simulink model "Orbit"  (R2019b)
settings: Solver=FixedStepAuto  StartTime=0.0  StopTime=24  RelTol=1e-3
InitFcn:
  | load('BusDefinitions.mat')
model workspace (MAT data in the model file):
  MM = [1  1  1  1; 1  1  -1  -1; 1  -1  -1  1; 1  -1  1  -1]
  OrbitLab = 0.5
  SlowDownPeriod = 3
  Startlag = 1
  initDesc = 20
  p = 0.8638671875
  wDotBias = 9.242
values from neighbouring files (symbols this model uses):
  A = double(subs(A4disc,9.81))    [loadDiscSys.m]
  At = A2by2    [KalmanGains.m]
  B = double(subs(B4disc,9.81))    [loadDiscSys.m]
  BMove = 11    [PrimeO.m]
  Bt = [0;-0.0624]    [KalmanGains.m]
  C = eye(2)    [KalmanGains.m]    (also in loadDiscSys.m = eye(4))
  commandZ = -1.5    [Commands.m]
  Ct = fsolve(hover,.05)    [BangBangCalculations.m]
  End = 13    [PrimeO.m]
  FMove = 9    [PrimeO.m]
  Ka = lqr(Aa,Ba,Qa,Ra)    [KalmanGains.m]
  KaI = Ka(1)/2    [Commands.m]
  Ke = lqr(Ae,Be,Qe,Re)    [KalmanGains.m]
  KeI = Ke(1)*1.5    [Commands.m]
  Kr = Kr    [KalmanGains.m]
  KrI = Kr(1)/4    [Commands.m]
  Kt = lqr(At,Bt,Qt,Rt)    [KalmanGains.m]
  KtI = Kt(1)/4    [Commands.m]
  LMove = 7    [PrimeO.m]
  R = eye(4)*.001    [KalmanCosts.m]
  RMove = 5    [PrimeO.m]
  Rt = 11    [KalmanCosts.m]    (also in KalmanGains.m = 0.005)
  tSwitch = fsolve(Switch,.5)    [BangBangCalculations.m]
  tSwitchU = tSwitch+.30    [BangBangCalculations.m]
  w0 = fsolve(hover,300)    [BangBangCalculations.m]
  wD = fsolve(Down,300)    [BangBangCalculations.m]
  wU = fsolve(Up,300)    [BangBangCalculations.m]
undefined symbols (not defined in the file or in its folder): codertarget, DiscIntNeverNeededParam, Discrete, Dt, Time
libraries: simulink x14, ctrlSharedLib x2
settings Model: ExtModeTrigDuration=80  OrderedModelArguments=off  Creator=johnharry  LastModifiedBy=johnh
settings OptimizationCC: BlockReduction=off  DefaultParameterBehavior=Inlined  BufferReuse=off  PassReuseOutputArgsThreshold=0  MaxStackSize=64
settings DebuggingCC: ParameterTunabilityLossMsg=error  ArithmeticOperatorsInVariantConditions=warning
settings HardwareCC: ProdBitPerPointer=32  ProdBitPerSizeT=32  ProdBitPerPtrDiffT=32  ProdLargestAtomicInteger=Long  ProdWordSize=32  ProdHWDeviceType=ARM Compatible->ARM 9
settings SFSimCC: SimUseLocalCustomCode=off  MATLABDynamicMemAlloc=off
settings RTWCC: SystemTargetFile=ert.tlc  HardwareBoard=PARROT Mambo  TLCOptions="-aInlineSetEventsForThisBaseRateFcn=TLC_FALSE -aSuppressMultiTaskScheduler=TLC_FALSE   -aRateBasedStepFcn=1"  TemplateMakefile=ert_default_tmf  GenerateReport=on  RTWUseLocalCustomCode=off  Toolchain=Sourcery G++ Lite GNU Toolchain for Drones  LaunchReport=on
settings CodeAppCC: ForceParamTrailComments=on  OperatorAnnotations=on  StateflowObjectComments=on
settings ERTTargetCC: ERTCustomFileBanners=off  MatFileLogging=on  SupportContinuousTime=on  SupportNonInlinedSFcns=on  RemoveResetFunc=off  ModelStepFunctionPrototypeControlCompliant=off

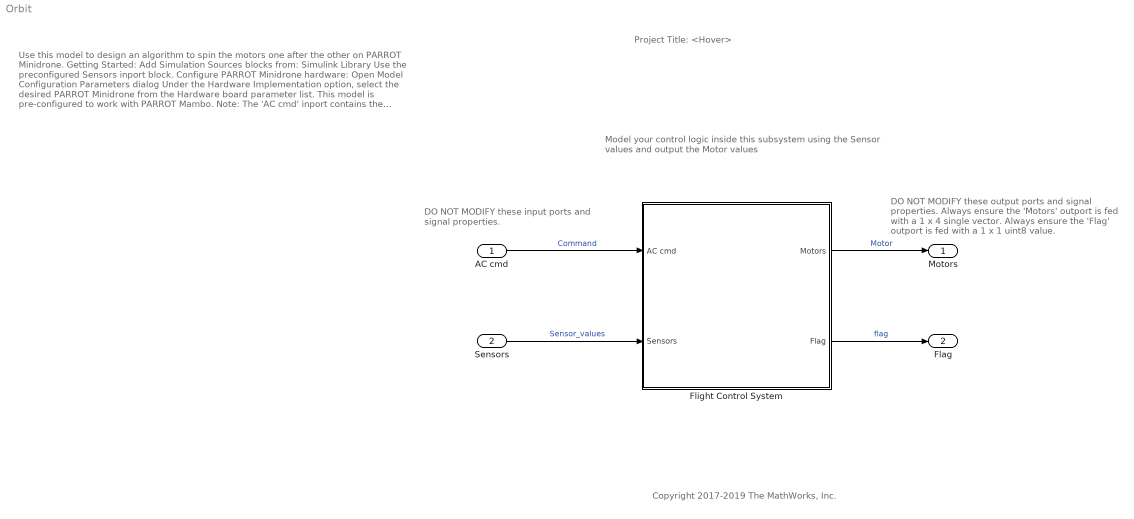
== system Orbit ==
  note: Model your control logic inside this subsystem
      | using the Sensor values and output the
      | Motor values
  note: DO NOT MODIFY these output ports
      | and signal properties.
      |
      |
      |
      | Always ensure the 'Motors' outport
      | is fed with a 1 x 4 single vector.
      |
      |
      |
      |
      |
      | Always ensure the 'Flag' outport is
      | fed with a 1 x 1 uint8 value.
  note: DO NOT MODIFY these input
      | ports and signal properties.
  note: Copyright 2017-2019 The MathWorks, Inc.
  note: Use this model to design an algorithm to spin the motors one
      | after the other on PARROT Minidrone.
      |
      | Getting Started:
      |
      | Add Simulation Sources blocks from:
      | Simulink Library
      | Use the preconfigured Sensors inport block.
      |
      | Configure PARROT Minidrone hardware:
      |
      | Open Model Configuration Parameters dialog
      |
      | Under the Hardware Implementation option, select the desired
      | PARROT Minidrone from the Hardware board parameter list.
      |
      | This model is pre-configured to work with PARROT Mambo.
      |
      | Note:
      |
      | The 'AC cmd' inport contains the position and orientation
      | reference signals information.
      | The 'Sensors' inport contains data from accelerometer,
      | gyroscope, ultrasonic, pressure and optical flow data.
      | The 'Flag' outport can be used to model an error condition
      | which stops the drone.
      | The 'Motors' outport is fed with the speed values of the 4 motors.
      | Learn more:
      |
      | Simulink Subsystem
      | Simulink Buses
  note: Project Title: <Hover>
  AC cmd : Inport  OutDataTypeStr=Bus: CommandBus  BusOutputAsStruct=on
  Sensors : Inport  Port=2  OutDataTypeStr=Bus: SensorsBus  BusOutputAsStruct=on
  Flight Control System : Subsystem  InitFcn=codertarget.parrot.internal.fcsSubsystemCallback(gcb);
  Motors : Outport  OutDataTypeStr=single  PortDimensions=[1 4]  VectorParamsAs1DForOutWhenUnconnected=off
  Flag : Outport  Port=2  OutDataTypeStr=uint8  PortDimensions=1  VectorParamsAs1DForOutWhenUnconnected=off
  wires:
  Flight Control System/1(Motors) -> Motors/1  "Motor"
  AC cmd/1 -> Flight Control System/1(AC cmd)  "Command"
  Sensors/1 -> Flight Control System/2(Sensors)  "Sensor_values"
  Flight Control System/2(Flag) -> Flag/1  "flag"

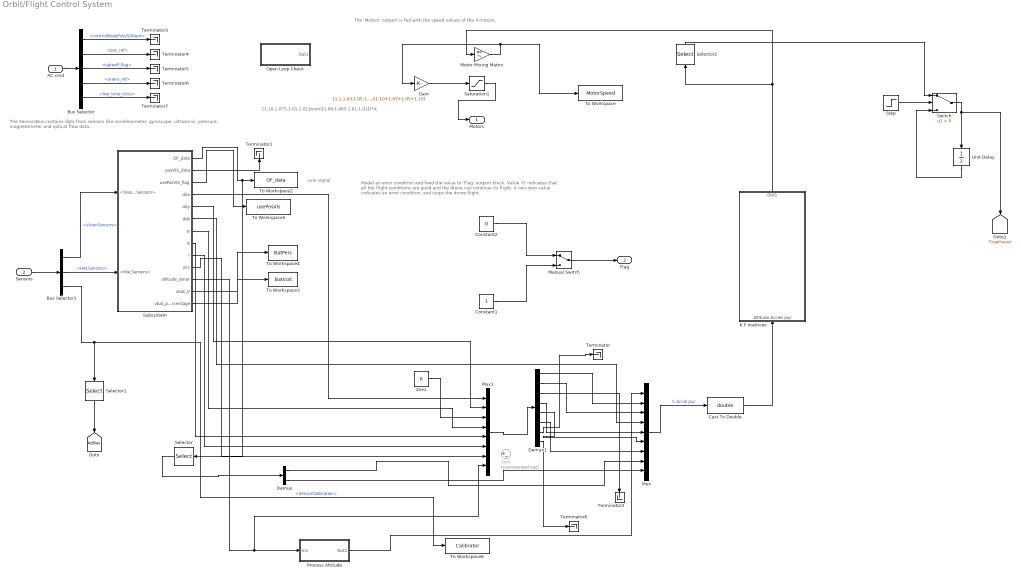
== system Orbit/Flight Control System ==
  note: [1.10,1.075,1.01,1.01]/sum([1.09,1.065,1.01,1.01])*4;
  note: uvw signal
  note: The 'Motors' outport is fed with the speed values of the 4 motors.
  note: Model an error condition and feed the value to 'Flag' outport block.
      | Value '0' indicates that all the flight conditions are good and the drone
      | can continue its flight.
      | A non-zero value indicates an error condition, and stops the drone
      | flight.
  note: The SensorsBus contains data from sensors like
      | accelerometer, gyroscope, ultrasonic, pressure,
      | magnetometer and optical flow data.
  AC cmd : Inport
  Sensors : Inport  Port=2
  Bus Selector : BusSelector  OutputSignals=controlModePosVSOrient,pos_ref,takeoff_flag,orient_ref,live_time_ticks
  Bus Selector1 : BusSelector  OutputSignals=VisionSensors,HALSensors,SensorCalibration
  Cast To Double : DataTypeConversion  OutDataTypeStr=double
  Constant1 : Constant  OutDataTypeStr=uint8
  Constant2 : Constant  Value=0  OutDataTypeStr=uint8
  Demux : Demux  Outputs=2
  Demux1 : Demux  Outputs=8
  Gain : Gain  Gain=[1.1,1.03,1.05,1.15].*4./(1.10+1.03+1.05+1.15)
  K F matrices : Subsystem
  Manual Switch : ManualSwitch
  Motor Mixing Matrix : Gain  Gain=MM  Multiplication=Matrix(K*u)
  Mux : Mux  Inputs=9
  Mux1 : Mux  Inputs=8
  Open Loop Check : Subsystem
  Process Altitude : Subsystem
  Saturation1 : Saturate  UpperLimit=500  LowerLimit=0  OutDataTypeStr=single
  Selector : Selector  InputPortWidth=3  IndexOptions=Index vector (dialog)  Indices=[1 2]  OutputSizes=1
  Selector1 : Selector  IndexOptions=Index vector (dialog)  Indices=3  OutputSizes=1
  Selector2 : Selector  InputPortWidth=4  IndexOptions=Index vector (dialog)  Indices=1  OutputSizes=1
  Step : Step  Time=tSwitch+tSwitchU+Startlag+OrbitLab  SampleTime=.005
  Subsystem : Subsystem
  Sum : Sum  Commented=on  Inputs=|+-
  Switch : Switch  Criteria=u2 > Threshold
  Terminator{,1..8} (9 alike) : Terminator
  To Workspace : ToWorkspace  VariableName=MotorSpeed  SaveFormat=Structure With Time  SampleTime=-1
  To Workspace2 : ToWorkspace  VariableName=OF_data  SaveFormat=Structure With Time  SampleTime=-1
  To Workspace3 : ToWorkspace  VariableName=BatVolt  SaveFormat=Structure With Time  SampleTime=-1
  To Workspace4 : ToWorkspace  VariableName=BatPerc  SaveFormat=Structure With Time  SampleTime=-1
  To Workspace5 : ToWorkspace  VariableName=usePosVis  SaveFormat=Structure With Time  SampleTime=-1
  To Workspace6 : ToWorkspace  VariableName=Calibrator  SaveFormat=Timeseries  SampleTime=-1
  Unit Delay : UnitDelay  SampleTime=-1  HasFrameUpgradeWarning=on
  Zero : Constant  Value=0  OutDataTypeStr=Inherit: Inherit via back propagation  SampleTime=.005
  Motors : Outport  VectorParamsAs1DForOutWhenUnconnected=off
  Flag : Outport  Port=2  VectorParamsAs1DForOutWhenUnconnected=off
  tag scope: AzBias=global, TrueHover=global
  wires:
  AC cmd/1 -> Bus Selector/1
  Sensors/1 -> Bus Selector1/1
  Bus Selector/1 -> Terminator3/1  "<controlModePosVSOrient>"
  Bus Selector/2 -> Terminator4/1  "<pos_ref>"
  Bus Selector/3 -> Terminator5/1  "<takeoff_flag>"
  Bus Selector/4 -> Terminator6/1  "<orient_ref>"
  Bus Selector/5 -> Terminator7/1  "<live_time_ticks>"
  Manual Switch/1 -> Flag/1
  Constant2/1 -> Manual Switch/1
  Constant1/1 -> Manual Switch/2
  Saturation1/1 -> Motors/1
  Bus Selector1/1 -> Subsystem/1(<VisionSensors>)  "<VisionSensors>"
  Bus Selector1/2 -> Subsystem/2(<HALSensors>)  "<HALSensors>"
  Bus Selector1/3 -> Selector1/1, To Workspace6/1  "<SensorCalibration>"
  Subsystem/1(OF_data) -> Selector/1, To Workspace2/1
  Subsystem/3(usePosVIS_flag) -> To Workspace5/1
  Subsystem/12(vbat_V) -> To Workspace3/1
  Subsystem/13(vbat_percentage) -> To Workspace4/1
  Subsystem/5(ddy) -> Mux1/2
  Subsystem/8(q) -> Mux1/5
  Subsystem/7(p) -> Mux1/4
  Subsystem/9(r) -> Mux1/6
  Subsystem/4(ddx) -> Mux1/1
  Mux/1 -> Cast To Double/1  "h Accel pqr"
  Subsystem/6(ddz) -> Mux/4
  Motor Mixing Matrix/1 -> Gain/1, To Workspace/1
  Subsystem/11(altitude_sonar) -> Mux1/8, Process Altitude/1(In1)
  K F matrices/1(Out1) -> Motor Mixing Matrix/1, Selector2/1
  Gain/1 -> Saturation1/1
  Cast To Double/1 -> K F matrices/1(Altitude Accels pqr)
  Selector/1 -> Demux/1
  Demux/1 -> Mux/8
  Demux/2 -> Mux/9
  Subsystem/10(prs) -> Mux1/7
  Mux1/1 -> Demux1/1
  Demux1/1 -> Mux/2
  Demux1/2 -> Mux/3
  Demux1/3 -> Terminator2/1
  Demux1/4 -> Mux/5
  Demux1/5 -> Mux/6
  Demux1/6 -> Mux/7
  Demux1/8 -> Terminator8/1
  Demux1/7 -> Terminator/1
  Subsystem/2(posVIS_data) -> Terminator1/1
  Zero/1 -> Mux1/3
  Selector1/1 -> [AzBias]
  Process Altitude/1(Out1) -> Mux/1
  Switch/1 -> [TrueHover], Unit Delay/1
  Selector2/1 -> Switch/1
  Unit Delay/1 -> Switch/3
  Step/1 -> Switch/2

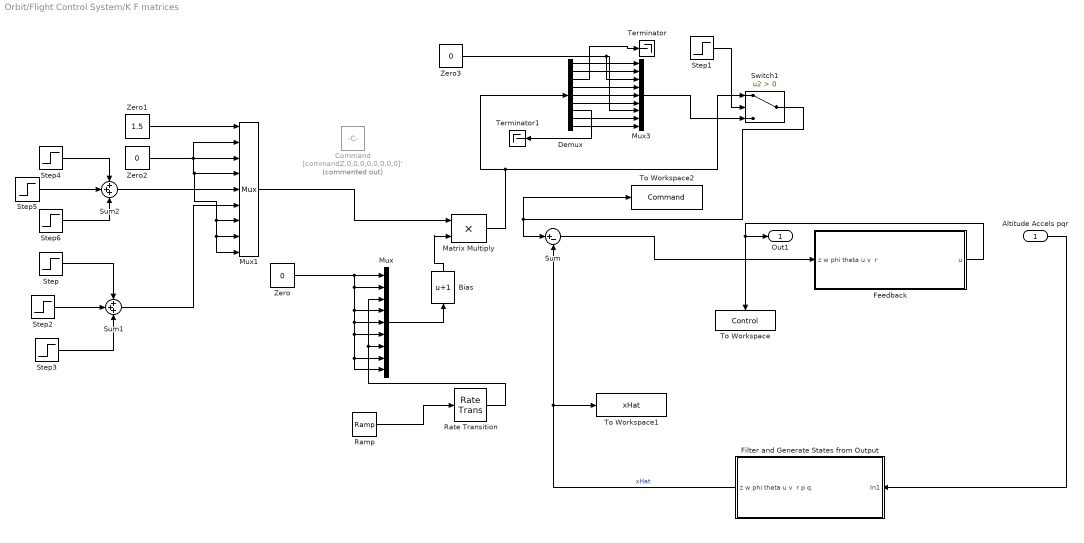
== system Orbit/Flight Control System/K F matrices ==
  Altitude Accels pqr : Inport
  Bias : Bias  Bias=1
  Command : Constant  Commented=on  Value=[commandZ,0,0,0,0,0,0,0,0]'  OutDataTypeStr=Inherit: Inherit via back propagation  SampleTime=.005
  Demux : Demux  Outputs=9
  Feedback : Subsystem
  Filter and Generate States from Output : Subsystem
  Matrix Multiply : Product
  Mux : Mux  Inputs=9
  Mux1 : Mux  Inputs=9
  Mux3 : Mux  Inputs=9
  Ramp : simulink/Sources/Ramp  slope=1/60  start=tSwitch+Startlag+tSwitchU+OrbitLab  InitialOutput=0
  Rate Transition : RateTransition  OutPortSampleTime=.005
  Step : Step  Time=RMove  After=.25  SampleTime=.005
  Step1 : Step  Time=initDesc-SlowDownPeriod  Before=1  After=-1  SampleTime=.005
  Step2 : Step  Time=LMove  After=-.5  SampleTime=.005
  Step3 : Step  Time=FMove  After=.25  SampleTime=.005
  Step4 : Step  Time=FMove  After=.25  SampleTime=.005
  Step5 : Step  Time=BMove  After=-.5  SampleTime=.005
  Step6 : Step  Time=End  After=.25  SampleTime=.005
  Sum : Sum  Inputs=|+-
  Sum1 : Sum  Inputs=+++
  Sum2 : Sum  Inputs=+++
  Switch1 : Switch  Criteria=u2 > Threshold
  Terminator : Terminator
  Terminator1 : Terminator
  To Workspace : ToWorkspace  VariableName=Control  SaveFormat=Structure With Time  SampleTime=-1
  To Workspace1 : ToWorkspace  VariableName=xHat  SaveFormat=Structure With Time  SampleTime=-1
  To Workspace2 : ToWorkspace  VariableName=Command  SaveFormat=Structure With Time  SampleTime=-1
  Zero : Constant  Value=0  OutDataTypeStr=Inherit: Inherit via back propagation  SampleTime=.005
  Zero1 : Constant  Value=1.5  OutDataTypeStr=Inherit: Inherit via back propagation  SampleTime=.005
  Zero2 : Constant  Value=0  OutDataTypeStr=Inherit: Inherit via back propagation  SampleTime=.005
  Zero3 : Constant  Value=0  OutDataTypeStr=Inherit: Inherit via back propagation  SampleTime=.005
  Out1 : Outport
  wires:
  Filter and Generate States from Output/1(z w phi theta u v  r p q) -> To Workspace1/1, Sum/2  "xHat"
  Feedback/1("u ") -> Out1/1, To Workspace/1
  Sum/1 -> Feedback/1(z w phi theta u v  r)
  Altitude Accels pqr/1 -> Filter and Generate States from Output/1(In1)
  Ramp/1 -> Rate Transition/1
  Rate Transition/1 -> Mux/3, Mux/7
  Zero/1 -> Mux/9, Mux/8, Mux/6, Mux/5, Mux/4, Mux/2, Mux/1
  Mux/1 -> Bias/1
  Bias/1 -> Matrix Multiply/2
  Matrix Multiply/1 -> Demux/1, Switch1/1
  Step1/1 -> Switch1/2
  Demux/1 -> Mux3/1
  Demux/2 -> Mux3/2
  Demux/9 -> Mux3/9
  Demux/8 -> Mux3/8
  Demux/7 -> Terminator1/1
  Demux/6 -> Mux3/6
  Demux/5 -> Mux3/5
  Demux/4 -> Mux3/4
  Mux3/1 -> Switch1/3
  Switch1/1 -> To Workspace2/1, Sum/1
  Zero3/1 -> Mux3/7, Mux3/3
  Demux/3 -> Terminator/1
  Zero1/1 -> Mux1/1
  Zero2/1 -> Mux1/8, Mux1/9, Mux1/7, Mux1/4, Mux1/3, Mux1/2
  Sum1/1 -> Mux1/6
  Sum2/1 -> Mux1/5
  Step3/1 -> Sum1/3
  Step2/1 -> Sum1/2
  Step/1 -> Sum1/1
  Step4/1 -> Sum2/1
  Step5/1 -> Sum2/2
  Step6/1 -> Sum2/3
  Mux1/1 -> Matrix Multiply/1

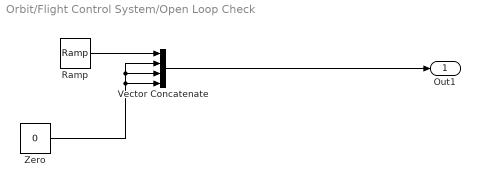
== system Orbit/Flight Control System/Open Loop Check ==
  Ramp : simulink/Sources/Ramp  slope=40  start=0  InitialOutput=0
  Vector Concatenate : Concatenate  NumInputs=4
  Zero : Constant  Value=0  OutDataTypeStr=Inherit: Inherit via back propagation
  Out1 : Outport
  wires:
  Vector Concatenate/1 -> Out1/1
  Zero/1 -> Vector Concatenate/4, Vector Concatenate/3, Vector Concatenate/2
  Ramp/1 -> Vector Concatenate/1

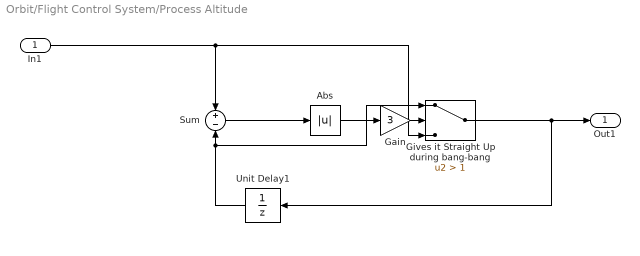
== system Orbit/Flight Control System/Process Altitude ==
  In1 : Inport  PortDimensions=1
  Abs : Abs
  Gain : Gain  Gain=3
  Gives it Straight Up during bang-bang : Switch  Criteria=u2 > Threshold  Threshold=1
  Sum : Sum  Inputs=+-
  Unit Delay1 : UnitDelay  SampleTime=-1  HasFrameUpgradeWarning=on
  Out1 : Outport  PortDimensions=1
  wires:
  In1/1 -> Gives it Straight Up during bang-bang/3, Sum/1
  Gives it Straight Up during bang-bang/1 -> Unit Delay1/1, Out1/1
  Unit Delay1/1 -> Gives it Straight Up during bang-bang/1, Sum/2
  Sum/1 -> Abs/1
  Abs/1 -> Gain/1
  Gain/1 -> Gives it Straight Up during bang-bang/2

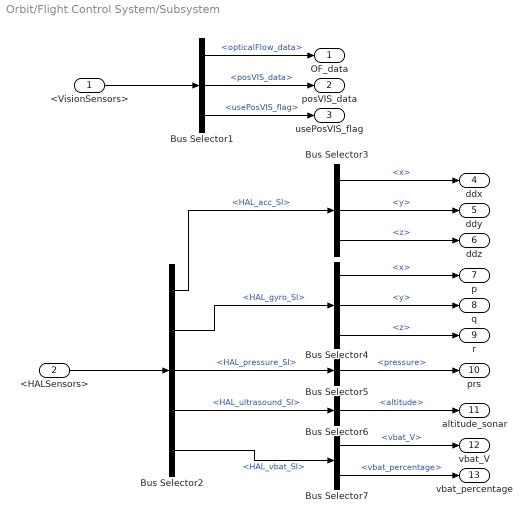
== system Orbit/Flight Control System/Subsystem ==
  <VisionSensors> : Inport
  <HALSensors> : Inport  Port=2
  Bus Selector1 : BusSelector  OutputSignals=opticalFlow_data,posVIS_data,usePosVIS_flag
  Bus Selector2 : BusSelector  OutputSignals=HAL_acc_SI,HAL_gyro_SI,HAL_pressure_SI,HAL_ultrasound_SI,HAL_vbat_SI
  Bus Selector3 : BusSelector  OutputSignals=x,y,z
  Bus Selector4 : BusSelector  OutputSignals=x,y,z
  Bus Selector5 : BusSelector  OutputSignals=pressure
  Bus Selector6 : BusSelector  OutputSignals=altitude
  Bus Selector7 : BusSelector  OutputSignals=vbat_V,vbat_percentage
  OF_data : Outport  VectorParamsAs1DForOutWhenUnconnected=off
  posVIS_data : Outport  Port=2  VectorParamsAs1DForOutWhenUnconnected=off
  usePosVIS_flag : Outport  Port=3  VectorParamsAs1DForOutWhenUnconnected=off
  ddx : Outport  Port=4  VectorParamsAs1DForOutWhenUnconnected=off
  ddy : Outport  Port=5  VectorParamsAs1DForOutWhenUnconnected=off
  ddz : Outport  Port=6  VectorParamsAs1DForOutWhenUnconnected=off
  p : Outport  Port=7  VectorParamsAs1DForOutWhenUnconnected=off
  q : Outport  Port=8  VectorParamsAs1DForOutWhenUnconnected=off
  r : Outport  Port=9  VectorParamsAs1DForOutWhenUnconnected=off
  prs : Outport  Port=10  VectorParamsAs1DForOutWhenUnconnected=off
  altitude_sonar : Outport  Port=11  VectorParamsAs1DForOutWhenUnconnected=off
  vbat_V : Outport  Port=12  VectorParamsAs1DForOutWhenUnconnected=off
  vbat_percentage : Outport  Port=13  VectorParamsAs1DForOutWhenUnconnected=off
  wires:
  <VisionSensors>/1 -> Bus Selector1/1
  <HALSensors>/1 -> Bus Selector2/1
  Bus Selector1/1 -> OF_data/1  "<opticalFlow_data>"
  Bus Selector1/2 -> posVIS_data/1  "<posVIS_data>"
  Bus Selector1/3 -> usePosVIS_flag/1  "<usePosVIS_flag>"
  Bus Selector2/1 -> Bus Selector3/1  "<HAL_acc_SI>"
  Bus Selector2/2 -> Bus Selector4/1  "<HAL_gyro_SI>"
  Bus Selector2/3 -> Bus Selector5/1  "<HAL_pressure_SI>"
  Bus Selector2/4 -> Bus Selector6/1  "<HAL_ultrasound_SI>"
  Bus Selector2/5 -> Bus Selector7/1  "<HAL_vbat_SI>"
  Bus Selector3/1 -> ddx/1  "<x>"
  Bus Selector3/2 -> ddy/1  "<y>"
  Bus Selector3/3 -> ddz/1  "<z>"
  Bus Selector4/2 -> q/1  "<y>"
  Bus Selector4/1 -> p/1  "<x>"
  Bus Selector4/3 -> r/1  "<z>"
  Bus Selector5/1 -> prs/1  "<pressure>"
  Bus Selector6/1 -> altitude_sonar/1  "<altitude>"
  Bus Selector7/1 -> vbat_V/1  "<vbat_V>"
  Bus Selector7/2 -> vbat_percentage/1  "<vbat_percentage>"

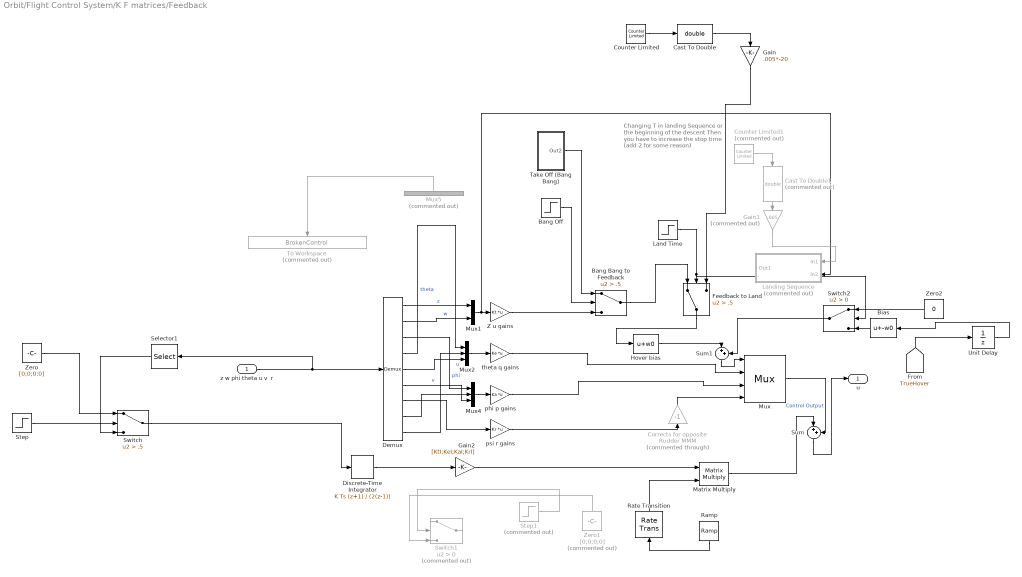
== system Orbit/Flight Control System/K F matrices/Feedback ==
  note: Changing T in landing Sequence
      | or the beginning of the descent
      | Then you have to increase the
      | stop time (add 2 for some reason)
  z w phi theta u v  r : Inport
  Bang Bang to Feedback : Switch  Criteria=u2 > Threshold  Threshold=.5
  "Bang Off " : Step  Time=Startlag+tSwitchU  Before=1  After=0  SampleTime=.005
  Bias : Bias  Bias=-w0
  Cast To Double : DataTypeConversion  OutDataTypeStr=double
  Cast To Double1 : DataTypeConversion  Commented=on  OutDataTypeStr=double
  Corrects for opposite Rudder MMM : Gain  Commented=through  Gain=-1
  Counter Limited : simulink/Sources/Counter Limited  uplimit=(initDesc-.005)*200  tsamp=.005
  Counter Limited1 : simulink/Sources/Counter Limited  Commented=on  uplimit=(initDesc-.005)*200  tsamp=.005
  Demux : Demux  Outputs=9
  Discrete-Time Integrator : DiscreteIntegrator  IntegratorMethod=Integration: Trapezoidal  SampleTime=-1  ICPrevOutput=DiscIntNeverNeededParam  ICPrevScaledInput=DiscIntNeverNeededParam
  Feedback to Land : Switch  Criteria=u2 > Threshold  Threshold=.5
  Gain : Gain  Gain=.005*-20
  Gain1 : Gain  Commented=on  Gain=.005
  Gain2 : Gain  Gain=[KtI;KeI;KaI;KrI]
  Hover bias : Bias  Bias=w0
  Land Time : Step  Time=initDesc  Before=1  After=0  SampleTime=.005
  Landing Sequence : Subsystem  Commented=on
  Matrix Multiply : Product  Multiplication=Matrix(*)
  Mux : Mux
  Mux1 : Mux  Inputs=2
  Mux2 : Mux  Inputs=3
  Mux4 : Mux  Inputs=3
  Mux5 : Mux  Commented=on  Inputs=8
  Ramp : simulink/Sources/Ramp  slope=-1/SlowDownPeriod  start=initDesc-SlowDownPeriod  InitialOutput=1
  Rate Transition : RateTransition  OutPortSampleTime=.005
  Selector1 : Selector  IndexOptions=Index vector (dialog)  Indices=[1 3 5 7]  OutputSizes=1
  Step : Step  Time=Startlag+tSwitchU  Before=1  After=0  SampleTime=.005
  Step1 : Step  Commented=on  Time=initDesc-2  Before=1  After=-1  SampleTime=.005
  Sum : Sum  Inputs=|++
  Sum1 : Sum  Inputs=|++
  Switch : Switch  Criteria=u2 > Threshold  Threshold=.5
  Switch1 : Switch  Commented=on  Criteria=u2 > Threshold
  Switch2 : Switch  Criteria=u2 > Threshold
  Take Off (Bang Bang) : Subsystem
  To Workspace : ToWorkspace  Commented=on  VariableName=BrokenControl  SaveFormat=Structure With Time  SampleTime=-1
  Unit Delay : UnitDelay  SampleTime=-1  HasFrameUpgradeWarning=on
  Z u gains : Gain  Gain=Kt  Multiplication=Matrix(K*u)
  Zero : Constant  Value=[0;0;0;0]  OutDataTypeStr=Inherit: Inherit via back propagation  SampleTime=.005
  Zero1 : Constant  Commented=on  Value=[0;0;0;0]  OutDataTypeStr=Inherit: Inherit via back propagation  SampleTime=.005
  Zero2 : Constant  Value=0  OutDataTypeStr=Inherit: Inherit via back propagation
  phi p gains : Gain  Gain=Ka  Multiplication=Matrix(K*u)
  psi r gains : Gain  Gain=Kr  Multiplication=Matrix(K*u)
  theta q gains : Gain  Gain=Ke  Multiplication=Matrix(K*u)
  "u " : Outport
  wires:
  Take Off (Bang Bang)/1(Out2) -> Bang Bang to Feedback/1
  Mux1/1 -> Landing Sequence/2(In2), Z u gains/1
  Z u gains/1 -> Bang Bang to Feedback/3
  Mux2/1 -> theta q gains/1
  psi r gains/1 -> Corrects for opposite Rudder MMM/1
  Mux4/1 -> phi p gains/1
  Mux/1 -> Sum/2  "Control Output"
  theta q gains/1 -> Mux/2
  phi p gains/1 -> Mux/3
  Corrects for opposite Rudder MMM/1 -> Mux/4
  z w phi theta u v  r/1 -> Selector1/1, Demux/1
  Bang Bang to Feedback/1 -> Feedback to Land/1
  Feedback to Land/1 -> Hover bias/1
  Mux5/1 -> To Workspace/1
  "Bang Off "/1 -> Bang Bang to Feedback/2
  Hover bias/1 -> Sum1/1
  Land Time/1 -> Switch2/2, Feedback to Land/2
  Demux/1 -> Mux1/1  "z"
  Demux/2 -> Mux1/2  "w"
  Demux/7 -> psi r gains/1
  Demux/6 -> Mux4/3  "v"
  Demux/5 -> Mux2/3  "u"
  Demux/3 -> Mux4/1  "phi"
  Demux/4 -> Mux2/1  "theta"
  Demux/8 -> Mux4/2
  Demux/9 -> Mux2/2
  Gain1/1 -> Landing Sequence/1(In1)
  Counter Limited/1 -> Cast To Double/1
  Cast To Double/1 -> Gain/1
  Counter Limited1/1 -> Cast To Double1/1
  Cast To Double1/1 -> Gain1/1
  Gain/1 -> Feedback to Land/3
  Sum/1 -> "u "/1
  Gain2/1 -> Matrix Multiply/1
  Discrete-Time Integrator/1 -> Gain2/1
  Step/1 -> Switch/2
  Zero/1 -> Switch/1
  Selector1/1 -> Switch/3
  Switch/1 -> Discrete-Time Integrator/1
  Step1/1 -> Switch1/2
  Zero1/1 -> Switch1/3
  Ramp/1 -> Rate Transition/1
  Matrix Multiply/1 -> Sum/1
  Rate Transition/1 -> Matrix Multiply/2
  Zero2/1 -> Switch2/1
  [TrueHover] -> Unit Delay/1
  Switch2/1 -> Sum1/2
  Bias/1 -> Switch2/3
  Sum1/1 -> Mux/1
  Unit Delay/1 -> Bias/1

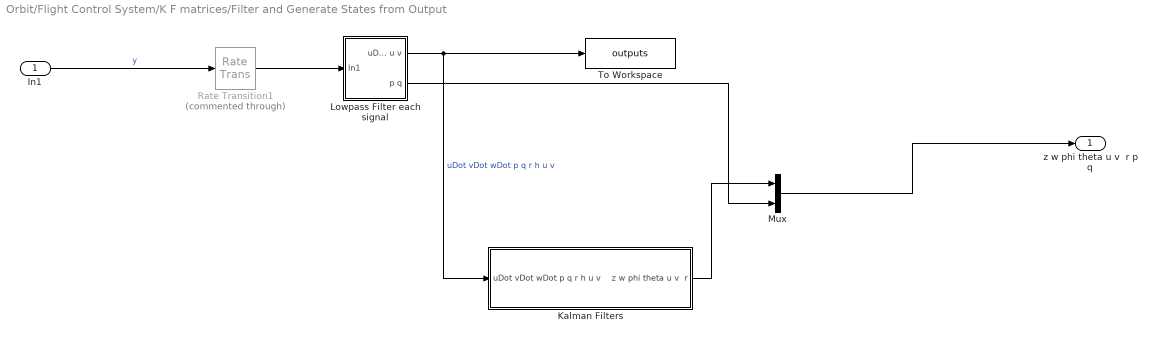
== system Orbit/Flight Control System/K F matrices/Filter and Generate States from Output ==
  In1 : Inport
  "Kalman Filters " : Subsystem
  Lowpass Filter each signal : Subsystem
  Mux : Mux  Inputs=2
  Rate Transition1 : RateTransition  Commented=through  OutPortSampleTime=.005
  To Workspace : ToWorkspace  VariableName=outputs  SaveFormat=Structure With Time  SampleTime=-1
  z w phi theta u v  r p q : Outport
  wires:
  In1/1 -> Rate Transition1/1  "y"
  "Kalman Filters "/1(z w phi theta u v  r) -> Mux/1
  Rate Transition1/1 -> Lowpass Filter each signal/1(In1)
  Lowpass Filter each signal/1(uDot vDot wDot p q r h u v) -> "Kalman Filters "/1(uDot vDot wDot p q r h u v), To Workspace/1  "uDot vDot wDot p q r h u v"
  Lowpass Filter each signal/2("p q ") -> Mux/2
  Mux/1 -> z w phi theta u v  r p q/1

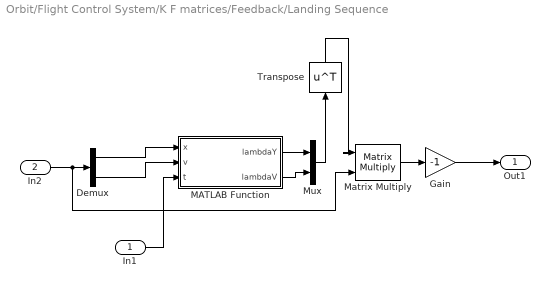
== system Orbit/Flight Control System/K F matrices/Feedback/Landing Sequence ==
  In1 : Inport
  In2 : Inport  Port=2
  Demux : Demux  Outputs=2
  Gain : Gain  Gain=-1
  MATLAB Function : MATLAB Function  TreatAsAtomicUnit=on
  Matrix Multiply : Product  Multiplication=Matrix(*)
  Mux : Mux  Inputs=2
  Transpose : Math  Operator=transpose  SignedPower=off  SaturateOnIntegerOverflow=on
  Out1 : Outport
  wires:
  In1/1 -> MATLAB Function/3(t)
  In2/1 -> Matrix Multiply/2, Demux/1
  Mux/1 -> Transpose/1
  MATLAB Function/1(lambdaY) -> Mux/1
  MATLAB Function/2(lambdaV) -> Mux/2
  Matrix Multiply/1 -> Gain/1
  Gain/1 -> Out1/1
  Demux/1 -> MATLAB Function/1(x)
  Demux/2 -> MATLAB Function/2(v)
  Transpose/1 -> Matrix Multiply/1

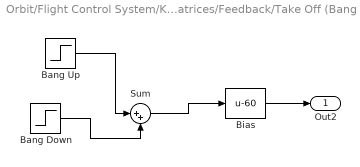
== system Orbit/Flight Control System/K F matrices/Feedback/Take Off (Bang Bang) ==
  Bang Down : Step  Time=Startlag+tSwitchU  After=wD-wU  SampleTime=.005
  Bang Up : Step  Time=Startlag  After=wU-w0+60  SampleTime=.005
  Bias : Bias  Bias=-60
  Sum : Sum  Inputs=|++
  Out2 : Outport
  wires:
  Bang Up/1 -> Sum/1
  Bang Down/1 -> Sum/2
  Sum/1 -> Bias/1
  Bias/1 -> Out2/1

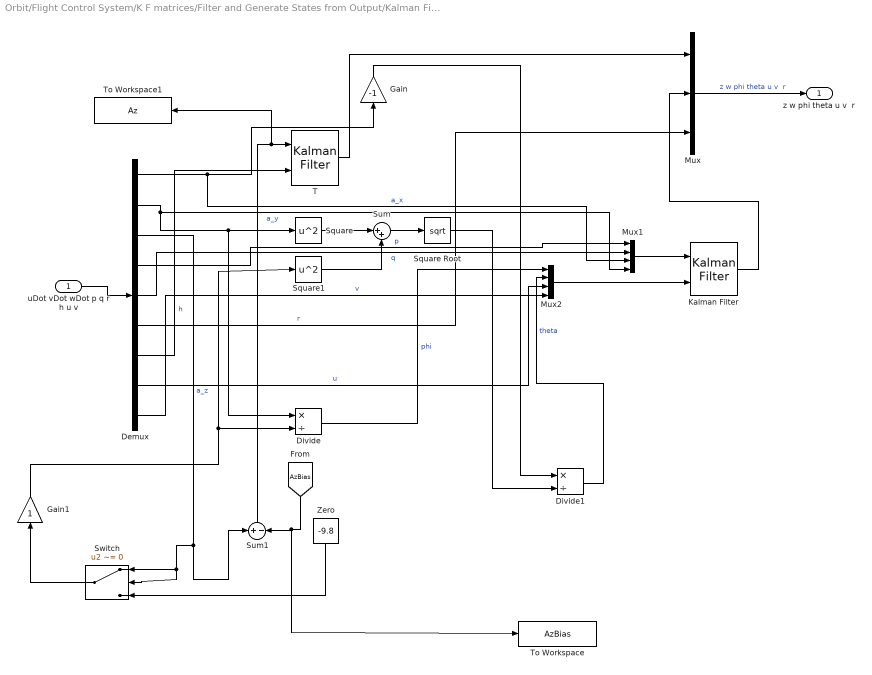
== system Orbit/Flight Control System/K F matrices/Filter and Generate States from Output/Kalman Filters  ==
  uDot vDot wDot p q r h u v : Inport
  Demux : Demux  Outputs=9
  Divide : Product  Inputs=*/
  Divide1 : Product  Inputs=*/
  Gain : Gain  Gain=-1
  Gain1 : Gain
  Kalman Filter : ctrlSharedLib/Kalman Filter  TimeDomain=Discrete-Time  UseCurrentEstimator=on  ModelSource=Individual A, B, C, D matrices  ModelSourceVariable=ss(0.95,1,1,0,1)  A=A  B=B  C=C  D=0  NumberOfStates=1  NumberOfInputs=1  NumberOfOutputs=1  InitialEstimateSource=Dialog  X0=0  P0=10  UseK=off  UseGH=off  NumberOfProcessNoiseInputs=1  G=1  TimeInvariantG=on  H=0  TimeInvariantH=on  Q=Q  TimeInvariantQ=on  R=R  TimeInvariantR=on  N=0  TimeInvariantN=on  AddInputPort=on  AddEnablePort=off  OutputEstimatedY=off  OutputP=off  Ts=-1
      settings: SourceProductBaseCode=CT
  Mux : Mux  Inputs=3
  Mux1 : Mux
  Mux2 : Mux
  Square : Math  Operator=square  SignedPower=off  SaturateOnIntegerOverflow=on
  Square Root : Sqrt  SaturateOnIntegerOverflow=on
  Square1 : Math  Operator=square  SignedPower=off  SaturateOnIntegerOverflow=on
  Sum : Sum  Inputs=|++
  Sum1 : Sum  Inputs=+-
  Switch : Switch  Criteria=u2 ~= 0  Threshold=1
  T : ctrlSharedLib/Kalman Filter  TimeDomain=Discrete-Time  UseCurrentEstimator=on  ModelSource=Individual A, B, C, D matrices  ModelSourceVariable=ss(At,Bt,Ct,Dt)  A=At  B=Bt  C=Ct  D=0  NumberOfStates=1  NumberOfInputs=1  NumberOfOutputs=1  InitialEstimateSource=Dialog  X0=[0;0]  P0=10  UseK=off  UseGH=off  NumberOfProcessNoiseInputs=1  G=1  TimeInvariantG=on  H=0  TimeInvariantH=on  Q=Qt  TimeInvariantQ=on  R=Rt  TimeInvariantR=on  N=0  TimeInvariantN=on  AddInputPort=on  AddEnablePort=off  OutputEstimatedY=off  OutputP=off  Ts=.005
      settings: SourceProductBaseCode=CT
  To Workspace : ToWorkspace  VariableName=AzBias  SaveFormat=Structure With Time  SampleTime=-1
  To Workspace1 : ToWorkspace  VariableName=Az  SaveFormat=Structure With Time  SampleTime=-1
  Zero : Constant  Value=-9.8  OutDataTypeStr=Inherit: Inherit via back propagation  SampleTime=.005
  z w phi theta u v  r : Outport
  wires:
  Sum/1 -> Square Root/1
  Demux/9 -> Mux2/4  "v"
  Square Root/1 -> Divide1/2
  Demux/4 -> Mux1/1  "p"
  Gain/1 -> Divide1/1
  Square1/1 -> Sum/2
  Square/1 -> Sum/1
  Divide1/1 -> Mux2/2  "theta"
  T/1 -> Mux/1
  Divide/1 -> Mux2/1  "phi"
  Mux/1 -> z w phi theta u v  r/1  "z w phi theta u v  r"
  uDot vDot wDot p q r h u v/1 -> Demux/1
  Demux/8 -> Mux2/3  "u"
  Demux/5 -> Mux1/2  "q"
  Demux/7 -> T/2  "h"
  Demux/2 -> Divide/1, Square/1, Mux1/4  "a_y"
  Demux/1 -> Mux1/3, Gain/1  "a_x"
  Demux/6 -> Mux/3  "r"
  Demux/3 -> Sum1/1, Switch/2, Switch/1  "a_z"
  Zero/1 -> Switch/3
  Sum1/1 -> To Workspace1/1, T/1
  Mux1/1 -> Kalman Filter/1
  Mux2/1 -> Kalman Filter/2
  Kalman Filter/1 -> Mux/2
  [AzBias] -> To Workspace/1, Sum1/2
  Switch/1 -> Gain1/1
  Gain1/1 -> Square1/1, Divide/2

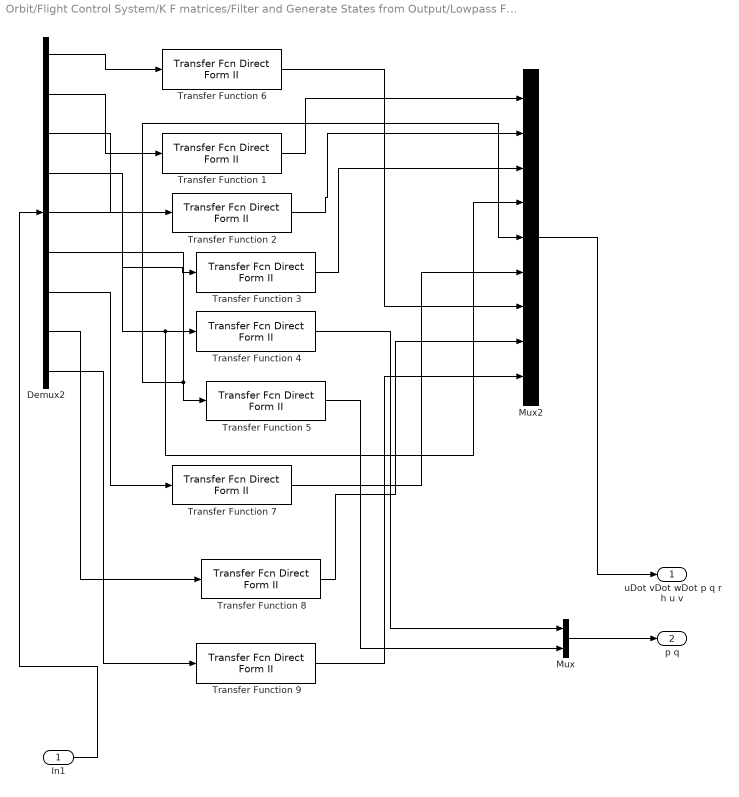
== system Orbit/Flight Control System/K F matrices/Filter and Generate States from Output/Lowpass Filter each signal ==
  In1 : Inport
  Demux2 : Demux  Outputs=9
  Mux : Mux  Inputs=2
  Mux2 : Mux  Inputs=9
  Transfer Function {1..6,8..9} (8 alike) : simulink/Additional Math & Discrete/Additional Discrete/Transfer Fcn Direct Form II  NumCoefVec=num  DenCoefVec=denom  vinit=0.0  DoSatur=off
      settings: SourceProductName=Simulink  SourceProductBaseCode=SL
  Transfer Function 7 : simulink/Additional Math & Discrete/Additional Discrete/Transfer Fcn Direct Form II  NumCoefVec=rnum  DenCoefVec=rdenom  vinit=0.0  DoSatur=off
      settings: SourceProductName=Simulink  SourceProductBaseCode=SL
  uDot vDot wDot p q r h u v : Outport
  "p q " : Outport  Port=2
  wires:
  Demux2/4 -> Transfer Function 3/1
  Transfer Function 1/1 -> Mux2/1
  Transfer Function 4/1 -> Mux/1
  Transfer Function 6/1 -> Mux2/7
  Transfer Function 3/1 -> Mux2/3
  Demux2/5 -> Mux2/4, Transfer Function 4/1
  Demux2/2 -> Transfer Function 1/1
  Transfer Function 2/1 -> Mux2/2
  Demux2/1 -> Transfer Function 6/1
  Demux2/3 -> Transfer Function 2/1
  Demux2/6 -> Mux2/5, Transfer Function 5/1
  Mux2/1 -> uDot vDot wDot p q r h u v/1
  In1/1 -> Demux2/1
  Transfer Function 5/1 -> Mux/2
  Demux2/7 -> Transfer Function 7/1
  Transfer Function 7/1 -> Mux2/6
  Demux2/8 -> Transfer Function 8/1
  Transfer Function 8/1 -> Mux2/8
  Demux2/9 -> Transfer Function 9/1
  Transfer Function 9/1 -> Mux2/9
  Mux/1 -> "p q "/1

== matlab function Orbit/Flight Control System/K F matrices/Feedback/Landing Sequence/MATLAB Function ==
  data: x input; v input; lambdaY output; t input; lambdaV output
function [lambdaY,lambdaV] = fcn(x,v,t)
c1=1;
c2=15;
T=2;
D = @(t,c2,c3)  (1/c2+1/3*(x)^3)*(1/c1+x)-1/4*x^4;
lambdaV = (1/c2+1/c1*(T-t)^2+1/3*(T-t)^3)/D(T-t,c1,c2);
lambdaY = (1/c1*(T-t)+1/2*(T-t)^2)/D(T-t,c1,c2);
if t>T
    lambdaV =0;
    lambdaY=0;
end 
end
